simulink model "ALL_JP360_DBW_V6_5_1103"  (R2022a)
settings: Solver=FixedStepAuto  StartTime=0.0  StopTime=inf  FixedStep=0.01  RelTol=1e-3  EnableMultiTasking=on
model workspace (MAT data in the model file):
  g = 9.8
undefined symbols (not defined in the file or in its folder): canChannel, delta_v_p, IPM_Line_C0, IPM_Line_C1, IPM_Line_C2, IPM_Line_C3, M, M_p, MRR_ObjDistX, MRR_ObjDistY, MRR_ObjFusionCamID, MRR_ObjFusionSig, MRR_ObjID, MRR_ObjRelVelX, MRR_ObjRelVelY, MRR_ObjType, MRR_ObjUpdFlg, none, obj_vaild, untracktime, V, videoinput
libraries: canfdmsglib x230, canfdlib x76, slpidlib x24, simulink x18, dspstat3 x14, ctrlSharedLib x1, simulink_extras x1, imaqlib x1, realtime_pacer_lib x1, dspvision x1, visionsinks x1
(part 46 of 55)

== system ALL_JP360_DBW_V6_5_1103/MsgFromCAN/VR_ADCU_MsgFromCAN/VR_ADCU_MRR_ObjHeader_0x680 ==
  VR_ADCU_MRR_ObjHeader_0x680FromInData : Inport  OutDataTypeStr=Bus:CAN_FD_MESSAGE_BUS
  Bus Creator : BusCreator  Inputs=9  OutDataTypeStr=Bus:VR_ADCU_MRR_ObjHeader_0x680  NonVirtualBus=on
  CAN FD Unpack : canfdmsglib/CAN FD Unpack  CANdbFile=HiFire_T360_P789_1R1V_Pri_Matrix_CAN_V2.3_20220810.dbc  MsgList=(none)  MsgName=MRR_ObjHeader_0x680  ProtocolMode=CAN FD  MsgIDType=Standard (11-bit identifier)  MsgIdentifier=1664  MsgLength=20  SignalInfo={'MRR_AlignmentFail','6','1','BE','unsigned','Standard','0','1','0','0','1';'MRR_Calib_State','5','1','BE','unsigned','Standard','0','1','0','0','1';'MRR_HWFail','7','1','BE','unsigned','Standard','0','1','0','0','1';'MRR_ObjHeader_CRC','152','16','BE','unsigned','Standard','0','1','0','0','65535';'MRR_ObjHeader_MsgCounter','136','4','BE','unsigned','Standard','0','1','0','0','15';'MRR_Obj_TimeStampStatus','72','8','BE','unsigned','Standard','0','1','0','0','255';'MRR_Obj_TimeStamp_Nsec','66','30','BE','unsigned','Standard','0','1','0','0','1073741823';'MRR_Obj_TimeStamp_sec','32','32','BE','unsigned','Standard','0','1','0','0','4294967295';'MRR_Sensor_Dirty','4','1','BE','unsigned','Standard','0','1','0','0','1'}  IDPort=off  TimestampPort=off  ErrorPort=off  RemotePort=off  LengthPort=off  StatusPort=off  BRSPort=off  ESIPort=off  DLCPort=off  ApplyMinMax=off
      settings: SourceProductBaseCode=ME,XP,VN  DataFormat=CANdb specified signals
  Data Type Conversion{1..3,9} (4 alike) : DataTypeConversion  OutDataTypeStr=boolean  SaturateOnIntegerOverflow=off  RndMeth=Floor
  Data Type Conversion4 : DataTypeConversion  OutDataTypeStr=uint16  SaturateOnIntegerOverflow=off  RndMeth=Floor
  Data Type Conversion5 : DataTypeConversion  OutDataTypeStr=int8  SaturateOnIntegerOverflow=off  RndMeth=Floor
  Data Type Conversion6 : DataTypeConversion  OutDataTypeStr=uint8  SaturateOnIntegerOverflow=off  RndMeth=Floor
  Data Type Conversion7 : DataTypeConversion  OutDataTypeStr=int32  SaturateOnIntegerOverflow=off  RndMeth=Floor
  Data Type Conversion8 : DataTypeConversion  OutDataTypeStr=uint32  SaturateOnIntegerOverflow=off  RndMeth=Floor
  VR_ADCU_MRR_ObjHeader_0x680FromOutData : Outport  OutDataTypeStr=Bus:VR_ADCU_MRR_ObjHeader_0x680
  wires:
  CAN FD Unpack/1 -> Data Type Conversion1/1
  CAN FD Unpack/2 -> Data Type Conversion2/1
  CAN FD Unpack/3 -> Data Type Conversion3/1
  CAN FD Unpack/4 -> Data Type Conversion4/1
  CAN FD Unpack/5 -> Data Type Conversion5/1
  CAN FD Unpack/6 -> Data Type Conversion6/1
  CAN FD Unpack/7 -> Data Type Conversion7/1
  CAN FD Unpack/8 -> Data Type Conversion8/1
  CAN FD Unpack/9 -> Data Type Conversion9/1
  Data Type Conversion1/1 -> Bus Creator/1  "MRR_AlignmentFail"
  Data Type Conversion2/1 -> Bus Creator/2  "MRR_Calib_State"
  Data Type Conversion3/1 -> Bus Creator/3  "MRR_HWFail"
  Data Type Conversion4/1 -> Bus Creator/4  "MRR_ObjHeader_CRC"
  Data Type Conversion5/1 -> Bus Creator/5  "MRR_ObjHeader_MsgCounter"
  Data Type Conversion6/1 -> Bus Creator/6  "MRR_Obj_TimeStampStatus"
  Data Type Conversion7/1 -> Bus Creator/7  "MRR_Obj_TimeStamp_Nsec"
  Data Type Conversion8/1 -> Bus Creator/8  "MRR_Obj_TimeStamp_sec"
  Data Type Conversion9/1 -> Bus Creator/9  "MRR_Sensor_Dirty"
  Bus Creator/1 -> VR_ADCU_MRR_ObjHeader_0x680FromOutData/1  "VR_ADCU_MRR_ObjHeader_0x680FromOutData"
  VR_ADCU_MRR_ObjHeader_0x680FromInData/1 -> CAN FD Unpack/1  "VR_ADCU_MRR_ObjHeader_0x680FromInData"

== system ALL_JP360_DBW_V6_5_1103/MsgFromCAN/VR_ADCU_MsgFromCAN/VR_ADCU_MRR_Obj_01_02_0x690 ==
  VR_ADCU_MRR_Obj_01_02_0x690FromInData : Inport  OutDataTypeStr=Bus:CAN_FD_MESSAGE_BUS
  Bus Creator : BusCreator  Inputs=30  OutDataTypeStr=Bus:VR_ADCU_MRR_Obj_01_02_0x690  NonVirtualBus=on
  CAN FD Unpack : canfdmsglib/CAN FD Unpack  CANdbFile=HiFire_T360_P789_1R1V_Pri_Matrix_CAN_V2.3_20220810.dbc  MsgList=(none)  MsgName=MRR_Obj_01_02_0x690  ProtocolMode=CAN FD  MsgIDType=Standard (11-bit identifier)  MsgIdentifier=1680  MsgLength=32  SignalInfo={'MRR_ObjDistX_01','26','12','BE','unsigned','Standard','0','0.0625','0','0','254.9375';'MRR_ObjDistX_02','130','12','BE','unsigned','Standard','0','0.0625','0','0','254.9375';'MRR_ObjDistY_01','44','14','BE','unsigned','Standard','0','0.0078125','-64','-64','63.9922';'MRR_ObjDistY_02','148','14','BE','unsigned','Standard','0','0.0078125','-64','-64','63.9922';'MRR_ObjExistProb_01','11','5','BE','unsigned','Standard','0','0.03125','0','0','0.96875';'MRR_ObjExistProb_02','115','5','BE','unsigned','Standard','0','0.03125','0','0','0.96875';'MRR_ObjFusionCamID_01','208','8','BE','unsigned','Standard','0','1','0','0','255';'MRR_ObjFusionCamID_02','216','8','BE','unsigned','Standard','0','1','0','0','255';'MRR_ObjFusionSig_01','98','2','BE','unsigned','Standard','0','1','0','0','3';'MRR_ObjFusionSig_02','202','2','BE','unsigned','Standard','0','1','0','0','3';'MRR_ObjID_01','0','8','BE','unsigned','Standard','0','1','0','0','255';'MRR_ObjID_02','104','8','BE','unsigned','Standard','0','1','0','0','255';'MRR_ObjMovingSts_01','103','3','BE','unsigned','Standard','0','1','0','0','7';'MRR_ObjMovingSts_02','207','3','BE','unsigned','Standard','0','1','0','0','7';'MRR_ObjObstacleProb_01','22','5','BE','unsigned','Standard','0','0.03125','0','0','0.96875';'MRR_ObjObstacleProb_02','126','5','BE','unsigned','Standard','0','0.03125','0','0','0.96875';'MRR_ObjRelAccelX_01','72','10','BE','unsigned','Standard','0','0.03125','-16','-16','15.9688';'MRR_ObjRelAccelX_02','176','10','BE','unsigned','Standard','0','0.03125','-16','-16','15.9688';'MRR_ObjRelAccelY_01','94','10','BE','unsigned','Standard','0','0.03125','-16','-16','15.9688';'MRR_ObjRelAccelY_02','198','10','BE','unsigned','Standard','0','0.03125','-16','-16','15.9688';'MRR_ObjRelVelX_01','63','13','BE','unsigned','Standard','0','0.03125','-128','-128','127.9688';'MRR_ObjRelVelX_02','167','13','BE','unsigned','Standard','0','0.03125','-128','-128','127.9688';'MRR_ObjRelVelY_01','66','13','BE','unsigned','Standard','0','0.03125','-128','-128','127.9688';'MRR_ObjRelVelY_02','170','13','BE','unsigned','Standard','0','0.03125','-128','-128','127.9688';'MRR_ObjType_01','90','4','BE','unsigned','Standard','0','1','0','0','15';'MRR_ObjType_02','194','4','BE','unsigned','Standard','0','1','0','0','15';'MRR_ObjUpdFlg_01','100','3','BE','unsigned','Standard','0','1','0','0','7';'MRR_ObjUpdFlg_02','204','3','BE','unsigned','Standard','0','1','0','0','7';'MRR_Obj_01_02_Checksum','248','16','BE','unsigned','Standard','0','1','0','0','65535';'MRR_Obj_01_02_MsgCounter','232','4','BE','unsigned','Standard','0','1','0','0','15'}  IDPort=off  TimestampPort=off  ErrorPort=off  RemotePort=off  LengthPort=off  StatusPort=off  BRSPort=off  ESIPort=off  DLCPort=off  ApplyMinMax=off
      settings: SourceProductBaseCode=ME,XP,VN  DataFormat=CANdb specified signals
  Data Type Conversion{1..6,15..24} (16 alike) : DataTypeConversion  OutDataTypeStr=single  SaturateOnIntegerOverflow=off  RndMeth=Floor
  Data Type Conversion{9..10,13..14,25..28,30} (9 alike) : DataTypeConversion  OutDataTypeStr=int8  SaturateOnIntegerOverflow=off  RndMeth=Floor
  Data Type Conversion{7..8,11..12} (4 alike) : DataTypeConversion  OutDataTypeStr=uint8  SaturateOnIntegerOverflow=off  RndMeth=Floor
  Data Type Conversion29 : DataTypeConversion  OutDataTypeStr=uint16  SaturateOnIntegerOverflow=off  RndMeth=Floor
  VR_ADCU_MRR_Obj_01_02_0x690FromOutData : Outport  OutDataTypeStr=Bus:VR_ADCU_MRR_Obj_01_02_0x690
  wires:
  CAN FD Unpack/1 -> Data Type Conversion1/1
  CAN FD Unpack/2 -> Data Type Conversion2/1
  CAN FD Unpack/3 -> Data Type Conversion3/1
  CAN FD Unpack/4 -> Data Type Conversion4/1
  CAN FD Unpack/5 -> Data Type Conversion5/1
  CAN FD Unpack/6 -> Data Type Conversion6/1
  CAN FD Unpack/7 -> Data Type Conversion7/1
  CAN FD Unpack/8 -> Data Type Conversion8/1
  CAN FD Unpack/9 -> Data Type Conversion9/1
  CAN FD Unpack/10 -> Data Type Conversion10/1
  CAN FD Unpack/11 -> Data Type Conversion11/1
  CAN FD Unpack/12 -> Data Type Conversion12/1
  CAN FD Unpack/13 -> Data Type Conversion13/1
  CAN FD Unpack/14 -> Data Type Conversion14/1
  CAN FD Unpack/15 -> Data Type Conversion15/1
  CAN FD Unpack/16 -> Data Type Conversion16/1
  CAN FD Unpack/17 -> Data Type Conversion17/1
  CAN FD Unpack/18 -> Data Type Conversion18/1
  CAN FD Unpack/19 -> Data Type Conversion19/1
  CAN FD Unpack/20 -> Data Type Conversion20/1
  CAN FD Unpack/21 -> Data Type Conversion21/1
  CAN FD Unpack/22 -> Data Type Conversion22/1
  CAN FD Unpack/23 -> Data Type Conversion23/1
  CAN FD Unpack/24 -> Data Type Conversion24/1
  CAN FD Unpack/25 -> Data Type Conversion25/1
  CAN FD Unpack/26 -> Data Type Conversion26/1
  CAN FD Unpack/27 -> Data Type Conversion27/1
  CAN FD Unpack/28 -> Data Type Conversion28/1
  CAN FD Unpack/29 -> Data Type Conversion29/1
  CAN FD Unpack/30 -> Data Type Conversion30/1
  Data Type Conversion1/1 -> Bus Creator/1  "MRR_ObjDistX_01"
  Data Type Conversion2/1 -> Bus Creator/2  "MRR_ObjDistX_02"
  Data Type Conversion3/1 -> Bus Creator/3  "MRR_ObjDistY_01"
  Data Type Conversion4/1 -> Bus Creator/4  "MRR_ObjDistY_02"
  Data Type Conversion5/1 -> Bus Creator/5  "MRR_ObjExistProb_01"
  Data Type Conversion6/1 -> Bus Creator/6  "MRR_ObjExistProb_02"
  Data Type Conversion7/1 -> Bus Creator/7  "MRR_ObjFusionCamID_01"
  Data Type Conversion8/1 -> Bus Creator/8  "MRR_ObjFusionCamID_02"
  Data Type Conversion9/1 -> Bus Creator/9  "MRR_ObjFusionSig_01"
  Data Type Conversion10/1 -> Bus Creator/10  "MRR_ObjFusionSig_02"
  Data Type Conversion11/1 -> Bus Creator/11  "MRR_ObjID_01"
  Data Type Conversion12/1 -> Bus Creator/12  "MRR_ObjID_02"
  Data Type Conversion13/1 -> Bus Creator/13  "MRR_ObjMovingSts_01"
  Data Type Conversion14/1 -> Bus Creator/14  "MRR_ObjMovingSts_02"
  Data Type Conversion15/1 -> Bus Creator/15  "MRR_ObjObstacleProb_01"
  Data Type Conversion16/1 -> Bus Creator/16  "MRR_ObjObstacleProb_02"
  Data Type Conversion17/1 -> Bus Creator/17  "MRR_ObjRelAccelX_01"
  Data Type Conversion18/1 -> Bus Creator/18  "MRR_ObjRelAccelX_02"
  Data Type Conversion19/1 -> Bus Creator/19  "MRR_ObjRelAccelY_01"
  Data Type Conversion20/1 -> Bus Creator/20  "MRR_ObjRelAccelY_02"
  Data Type Conversion21/1 -> Bus Creator/21  "MRR_ObjRelVelX_01"
  Data Type Conversion22/1 -> Bus Creator/22  "MRR_ObjRelVelX_02"
  Data Type Conversion23/1 -> Bus Creator/23  "MRR_ObjRelVelY_01"
  Data Type Conversion24/1 -> Bus Creator/24  "MRR_ObjRelVelY_02"
  Data Type Conversion25/1 -> Bus Creator/25  "MRR_ObjType_01"
  Data Type Conversion26/1 -> Bus Creator/26  "MRR_ObjType_02"
  Data Type Conversion27/1 -> Bus Creator/27  "MRR_ObjUpdFlg_01"
  Data Type Conversion28/1 -> Bus Creator/28  "MRR_ObjUpdFlg_02"
  Data Type Conversion29/1 -> Bus Creator/29  "MRR_Obj_01_02_Checksum"
  Data Type Conversion30/1 -> Bus Creator/30  "MRR_Obj_01_02_MsgCounter"
  Bus Creator/1 -> VR_ADCU_MRR_Obj_01_02_0x690FromOutData/1  "VR_ADCU_MRR_Obj_01_02_0x690FromOutData"
  VR_ADCU_MRR_Obj_01_02_0x690FromInData/1 -> CAN FD Unpack/1  "VR_ADCU_MRR_Obj_01_02_0x690FromInData"

== system ALL_JP360_DBW_V6_5_1103/MsgFromCAN/VR_ADCU_MsgFromCAN/VR_ADCU_MRR_Obj_03_04_0x691 ==
  VR_ADCU_MRR_Obj_03_04_0x691FromInData : Inport  OutDataTypeStr=Bus:CAN_FD_MESSAGE_BUS
  Bus Creator : BusCreator  Inputs=30  OutDataTypeStr=Bus:VR_ADCU_MRR_Obj_03_04_0x691  NonVirtualBus=on
  CAN FD Unpack : canfdmsglib/CAN FD Unpack  CANdbFile=HiFire_T360_P789_1R1V_Pri_Matrix_CAN_V2.3_20220810.dbc  MsgList=(none)  MsgName=MRR_Obj_03_04_0x691  ProtocolMode=CAN FD  MsgIDType=Standard (11-bit identifier)  MsgIdentifier=1681  MsgLength=32  SignalInfo={'MRR_ObjDistX_03','26','12','BE','unsigned','Standard','0','0.0625','0','0','254.9375';'MRR_ObjDistX_04','130','12','BE','unsigned','Standard','0','0.0625','0','0','254.9375';'MRR_ObjDistY_03','44','14','BE','unsigned','Standard','0','0.0078125','-64','-64','63.9922';'MRR_ObjDistY_04','148','14','BE','unsigned','Standard','0','0.0078125','-64','-64','63.9922';'MRR_ObjExistProb_03','11','5','BE','unsigned','Standard','0','0.03125','0','0','0.96875';'MRR_ObjExistProb_04','115','5','BE','unsigned','Standard','0','0.03125','0','0','0.96875';'MRR_ObjFusionCamID_03','208','8','BE','unsigned','Standard','0','1','0','0','255';'MRR_ObjFusionCamID_04','216','8','BE','unsigned','Standard','0','1','0','0','255';'MRR_ObjFusionSig_03','98','2','BE','unsigned','Standard','0','1','0','0','3';'MRR_ObjFusionSig_04','202','2','BE','unsigned','Standard','0','1','0','0','3';'MRR_ObjID_03','0','8','BE','unsigned','Standard','0','1','0','0','255';'MRR_ObjID_04','104','8','BE','unsigned','Standard','0','1','0','0','255';'MRR_ObjMovingSts_03','103','3','BE','unsigned','Standard','0','1','0','0','7';'MRR_ObjMovingSts_04','207','3','BE','unsigned','Standard','0','1','0','0','7';'MRR_ObjObstacleProb_03','22','5','BE','unsigned','Standard','0','0.03125','0','0','0.96875';'MRR_ObjObstacleProb_04','126','5','BE','unsigned','Standard','0','0.03125','0','0','0.96875';'MRR_ObjRelAccelX_03','72','10','BE','unsigned','Standard','0','0.03125','-16','-16','15.9688';'MRR_ObjRelAccelX_04','176','10','BE','unsigned','Standard','0','0.03125','-16','-16','15.9688';'MRR_ObjRelAccelY_03','94','10','BE','unsigned','Standard','0','0.03125','-16','-16','15.9688';'MRR_ObjRelAccelY_04','198','10','BE','unsigned','Standard','0','0.03125','-16','-16','15.9688';'MRR_ObjRelVelX_03','63','13','BE','unsigned','Standard','0','0.03125','-128','-128','127.9688';'MRR_ObjRelVelX_04','167','13','BE','unsigned','Standard','0','0.03125','-128','-128','127.9688';'MRR_ObjRelVelY_03','66','13','BE','unsigned','Standard','0','0.03125','-128','-128','127.9688';'MRR_ObjRelVelY_04','170','13','BE','unsigned','Standard','0','0.03125','-128','-128','127.9688';'MRR_ObjType_03','90','4','BE','unsigned','Standard','0','1','0','0','15';'MRR_ObjType_04','194','4','BE','unsigned','Standard','0','1','0','0','15';'MRR_ObjUpdFlg_03','100','3','BE','unsigned','Standard','0','1','0','0','7';'MRR_ObjUpdFlg_04','204','3','BE','unsigned','Standard','0','1','0','0','7';'MRR_Obj_03_04_Checksum','248','16','BE','unsigned','Standard','0','1','0','0','65535';'MRR_Obj_03_04_MsgCounter','232','4','BE','unsigned','Standard','0','1','0','0','15'}  IDPort=off  TimestampPort=off  ErrorPort=off  RemotePort=off  LengthPort=off  StatusPort=off  BRSPort=off  ESIPort=off  DLCPort=off  ApplyMinMax=off
      settings: SourceProductBaseCode=ME,XP,VN  DataFormat=CANdb specified signals
  Data Type Conversion{1..6,15..24} (16 alike) : DataTypeConversion  OutDataTypeStr=single  SaturateOnIntegerOverflow=off  RndMeth=Floor
  Data Type Conversion{9..10,13..14,25..28,30} (9 alike) : DataTypeConversion  OutDataTypeStr=int8  SaturateOnIntegerOverflow=off  RndMeth=Floor
  Data Type Conversion{7..8,11..12} (4 alike) : DataTypeConversion  OutDataTypeStr=uint8  SaturateOnIntegerOverflow=off  RndMeth=Floor
  Data Type Conversion29 : DataTypeConversion  OutDataTypeStr=uint16  SaturateOnIntegerOverflow=off  RndMeth=Floor
  VR_ADCU_MRR_Obj_03_04_0x691FromOutData : Outport  OutDataTypeStr=Bus:VR_ADCU_MRR_Obj_03_04_0x691
  wires:
  CAN FD Unpack/1 -> Data Type Conversion1/1
  CAN FD Unpack/2 -> Data Type Conversion2/1
  CAN FD Unpack/3 -> Data Type Conversion3/1
  CAN FD Unpack/4 -> Data Type Conversion4/1
  CAN FD Unpack/5 -> Data Type Conversion5/1
  CAN FD Unpack/6 -> Data Type Conversion6/1
  CAN FD Unpack/7 -> Data Type Conversion7/1
  CAN FD Unpack/8 -> Data Type Conversion8/1
  CAN FD Unpack/9 -> Data Type Conversion9/1
  CAN FD Unpack/10 -> Data Type Conversion10/1
  CAN FD Unpack/11 -> Data Type Conversion11/1
  CAN FD Unpack/12 -> Data Type Conversion12/1
  CAN FD Unpack/13 -> Data Type Conversion13/1
  CAN FD Unpack/14 -> Data Type Conversion14/1
  CAN FD Unpack/15 -> Data Type Conversion15/1
  CAN FD Unpack/16 -> Data Type Conversion16/1
  CAN FD Unpack/17 -> Data Type Conversion17/1
  CAN FD Unpack/18 -> Data Type Conversion18/1
  CAN FD Unpack/19 -> Data Type Conversion19/1
  CAN FD Unpack/20 -> Data Type Conversion20/1
  CAN FD Unpack/21 -> Data Type Conversion21/1
  CAN FD Unpack/22 -> Data Type Conversion22/1
  CAN FD Unpack/23 -> Data Type Conversion23/1
  CAN FD Unpack/24 -> Data Type Conversion24/1
  CAN FD Unpack/25 -> Data Type Conversion25/1
  CAN FD Unpack/26 -> Data Type Conversion26/1
  CAN FD Unpack/27 -> Data Type Conversion27/1
  CAN FD Unpack/28 -> Data Type Conversion28/1
  CAN FD Unpack/29 -> Data Type Conversion29/1
  CAN FD Unpack/30 -> Data Type Conversion30/1
  Data Type Conversion1/1 -> Bus Creator/1  "MRR_ObjDistX_03"
  Data Type Conversion2/1 -> Bus Creator/2  "MRR_ObjDistX_04"
  Data Type Conversion3/1 -> Bus Creator/3  "MRR_ObjDistY_03"
  Data Type Conversion4/1 -> Bus Creator/4  "MRR_ObjDistY_04"
  Data Type Conversion5/1 -> Bus Creator/5  "MRR_ObjExistProb_03"
  Data Type Conversion6/1 -> Bus Creator/6  "MRR_ObjExistProb_04"
  Data Type Conversion7/1 -> Bus Creator/7  "MRR_ObjFusionCamID_03"
  Data Type Conversion8/1 -> Bus Creator/8  "MRR_ObjFusionCamID_04"
  Data Type Conversion9/1 -> Bus Creator/9  "MRR_ObjFusionSig_03"
  Data Type Conversion10/1 -> Bus Creator/10  "MRR_ObjFusionSig_04"
  Data Type Conversion11/1 -> Bus Creator/11  "MRR_ObjID_03"
  Data Type Conversion12/1 -> Bus Creator/12  "MRR_ObjID_04"
  Data Type Conversion13/1 -> Bus Creator/13  "MRR_ObjMovingSts_03"
  Data Type Conversion14/1 -> Bus Creator/14  "MRR_ObjMovingSts_04"
  Data Type Conversion15/1 -> Bus Creator/15  "MRR_ObjObstacleProb_03"
  Data Type Conversion16/1 -> Bus Creator/16  "MRR_ObjObstacleProb_04"
  Data Type Conversion17/1 -> Bus Creator/17  "MRR_ObjRelAccelX_03"
  Data Type Conversion18/1 -> Bus Creator/18  "MRR_ObjRelAccelX_04"
  Data Type Conversion19/1 -> Bus Creator/19  "MRR_ObjRelAccelY_03"
  Data Type Conversion20/1 -> Bus Creator/20  "MRR_ObjRelAccelY_04"
  Data Type Conversion21/1 -> Bus Creator/21  "MRR_ObjRelVelX_03"
  Data Type Conversion22/1 -> Bus Creator/22  "MRR_ObjRelVelX_04"
  Data Type Conversion23/1 -> Bus Creator/23  "MRR_ObjRelVelY_03"
  Data Type Conversion24/1 -> Bus Creator/24  "MRR_ObjRelVelY_04"
  Data Type Conversion25/1 -> Bus Creator/25  "MRR_ObjType_03"
  Data Type Conversion26/1 -> Bus Creator/26  "MRR_ObjType_04"
  Data Type Conversion27/1 -> Bus Creator/27  "MRR_ObjUpdFlg_03"
  Data Type Conversion28/1 -> Bus Creator/28  "MRR_ObjUpdFlg_04"
  Data Type Conversion29/1 -> Bus Creator/29  "MRR_Obj_03_04_Checksum"
  Data Type Conversion30/1 -> Bus Creator/30  "MRR_Obj_03_04_MsgCounter"
  Bus Creator/1 -> VR_ADCU_MRR_Obj_03_04_0x691FromOutData/1  "VR_ADCU_MRR_Obj_03_04_0x691FromOutData"
  VR_ADCU_MRR_Obj_03_04_0x691FromInData/1 -> CAN FD Unpack/1  "VR_ADCU_MRR_Obj_03_04_0x691FromInData"

== system ALL_JP360_DBW_V6_5_1103/MsgFromCAN/VR_ADCU_MsgFromCAN/VR_ADCU_MRR_Obj_05_06_0x692 ==
  VR_ADCU_MRR_Obj_05_06_0x692FromInData : Inport  OutDataTypeStr=Bus:CAN_FD_MESSAGE_BUS
  Bus Creator : BusCreator  Inputs=30  OutDataTypeStr=Bus:VR_ADCU_MRR_Obj_05_06_0x692  NonVirtualBus=on
  CAN FD Unpack : canfdmsglib/CAN FD Unpack  CANdbFile=HiFire_T360_P789_1R1V_Pri_Matrix_CAN_V2.3_20220810.dbc  MsgList=(none)  MsgName=MRR_Obj_05_06_0x692  ProtocolMode=CAN FD  MsgIDType=Standard (11-bit identifier)  MsgIdentifier=1682  MsgLength=32  SignalInfo={'MRR_ObjDistX_05','26','12','BE','unsigned','Standard','0','0.0625','0','0','254.9375';'MRR_ObjDistX_06','130','12','BE','unsigned','Standard','0','0.0625','0','0','254.9375';'MRR_ObjDistY_05','44','14','BE','unsigned','Standard','0','0.0078125','-64','-64','63.9922';'MRR_ObjDistY_06','148','14','BE','unsigned','Standard','0','0.0078125','-64','-64','63.9922';'MRR_ObjExistProb_05','11','5','BE','unsigned','Standard','0','0.03125','0','0','0.96875';'MRR_ObjExistProb_06','115','5','BE','unsigned','Standard','0','0.03125','0','0','0.96875';'MRR_ObjFusionCamID_05','208','8','BE','unsigned','Standard','0','1','0','0','255';'MRR_ObjFusionCamID_06','216','8','BE','unsigned','Standard','0','1','0','0','255';'MRR_ObjFusionSig_05','98','2','BE','unsigned','Standard','0','1','0','0','3';'MRR_ObjFusionSig_06','202','2','BE','unsigned','Standard','0','1','0','0','3';'MRR_ObjID_05','0','8','BE','unsigned','Standard','0','1','0','0','255';'MRR_ObjID_06','104','8','BE','unsigned','Standard','0','1','0','0','255';'MRR_ObjMovingSts_05','103','3','BE','unsigned','Standard','0','1','0','0','7';'MRR_ObjMovingSts_06','207','3','BE','unsigned','Standard','0','1','0','0','7';'MRR_ObjObstacleProb_05','22','5','BE','unsigned','Standard','0','0.03125','0','0','0.96875';'MRR_ObjObstacleProb_06','126','5','BE','unsigned','Standard','0','0.03125','0','0','0.96875';'MRR_ObjRelAccelX_05','72','10','BE','unsigned','Standard','0','0.03125','-16','-16','15.9688';'MRR_ObjRelAccelX_06','176','10','BE','unsigned','Standard','0','0.03125','-16','-16','15.9688';'MRR_ObjRelAccelY_05','94','10','BE','unsigned','Standard','0','0.03125','-16','-16','15.9688';'MRR_ObjRelAccelY_06','198','10','BE','unsigned','Standard','0','0.03125','-16','-16','15.9688';'MRR_ObjRelVelX_05','63','13','BE','unsigned','Standard','0','0.03125','-128','-128','127.9688';'MRR_ObjRelVelX_06','167','13','BE','unsigned','Standard','0','0.03125','-128','-128','127.9688';'MRR_ObjRelVelY_05','66','13','BE','unsigned','Standard','0','0.03125','-128','-128','127.9688';'MRR_ObjRelVelY_06','170','13','BE','unsigned','Standard','0','0.03125','-128','-128','127.9688';'MRR_ObjType_05','90','4','BE','unsigned','Standard','0','1','0','0','15';'MRR_ObjType_06','194','4','BE','unsigned','Standard','0','1','0','0','15';'MRR_ObjUpdFlg_05','100','3','BE','unsigned','Standard','0','1','0','0','7';'MRR_ObjUpdFlg_06','204','3','BE','unsigned','Standard','0','1','0','0','7';'MRR_Obj_05_06_Checksum','248','16','BE','unsigned','Standard','0','1','0','0','65535';'MRR_Obj_05_06_MsgCounter','232','4','BE','unsigned','Standard','0','1','0','0','15'}  IDPort=off  TimestampPort=off  ErrorPort=off  RemotePort=off  LengthPort=off  StatusPort=off  BRSPort=off  ESIPort=off  DLCPort=off  ApplyMinMax=off
      settings: SourceProductBaseCode=ME,XP,VN  DataFormat=CANdb specified signals
  Data Type Conversion{1..6,15..24} (16 alike) : DataTypeConversion  OutDataTypeStr=single  SaturateOnIntegerOverflow=off  RndMeth=Floor
  Data Type Conversion{9..10,13..14,25..28,30} (9 alike) : DataTypeConversion  OutDataTypeStr=int8  SaturateOnIntegerOverflow=off  RndMeth=Floor
  Data Type Conversion{7..8,11..12} (4 alike) : DataTypeConversion  OutDataTypeStr=uint8  SaturateOnIntegerOverflow=off  RndMeth=Floor
  Data Type Conversion29 : DataTypeConversion  OutDataTypeStr=uint16  SaturateOnIntegerOverflow=off  RndMeth=Floor
  VR_ADCU_MRR_Obj_05_06_0x692FromOutData : Outport  OutDataTypeStr=Bus:VR_ADCU_MRR_Obj_05_06_0x692
  wires:
  CAN FD Unpack/1 -> Data Type Conversion1/1
  CAN FD Unpack/2 -> Data Type Conversion2/1
  CAN FD Unpack/3 -> Data Type Conversion3/1
  CAN FD Unpack/4 -> Data Type Conversion4/1
  CAN FD Unpack/5 -> Data Type Conversion5/1
  CAN FD Unpack/6 -> Data Type Conversion6/1
  CAN FD Unpack/7 -> Data Type Conversion7/1
  CAN FD Unpack/8 -> Data Type Conversion8/1
  CAN FD Unpack/9 -> Data Type Conversion9/1
  CAN FD Unpack/10 -> Data Type Conversion10/1
  CAN FD Unpack/11 -> Data Type Conversion11/1
  CAN FD Unpack/12 -> Data Type Conversion12/1
  CAN FD Unpack/13 -> Data Type Conversion13/1
  CAN FD Unpack/14 -> Data Type Conversion14/1
  CAN FD Unpack/15 -> Data Type Conversion15/1
  CAN FD Unpack/16 -> Data Type Conversion16/1
  CAN FD Unpack/17 -> Data Type Conversion17/1
  CAN FD Unpack/18 -> Data Type Conversion18/1
  CAN FD Unpack/19 -> Data Type Conversion19/1
  CAN FD Unpack/20 -> Data Type Conversion20/1
  CAN FD Unpack/21 -> Data Type Conversion21/1
  CAN FD Unpack/22 -> Data Type Conversion22/1
  CAN FD Unpack/23 -> Data Type Conversion23/1
  CAN FD Unpack/24 -> Data Type Conversion24/1
  CAN FD Unpack/25 -> Data Type Conversion25/1
  CAN FD Unpack/26 -> Data Type Conversion26/1
  CAN FD Unpack/27 -> Data Type Conversion27/1
  CAN FD Unpack/28 -> Data Type Conversion28/1
  CAN FD Unpack/29 -> Data Type Conversion29/1
  CAN FD Unpack/30 -> Data Type Conversion30/1
  Data Type Conversion1/1 -> Bus Creator/1  "MRR_ObjDistX_05"
  Data Type Conversion2/1 -> Bus Creator/2  "MRR_ObjDistX_06"
  Data Type Conversion3/1 -> Bus Creator/3  "MRR_ObjDistY_05"
  Data Type Conversion4/1 -> Bus Creator/4  "MRR_ObjDistY_06"
  Data Type Conversion5/1 -> Bus Creator/5  "MRR_ObjExistProb_05"
  Data Type Conversion6/1 -> Bus Creator/6  "MRR_ObjExistProb_06"
  Data Type Conversion7/1 -> Bus Creator/7  "MRR_ObjFusionCamID_05"
  Data Type Conversion8/1 -> Bus Creator/8  "MRR_ObjFusionCamID_06"
  Data Type Conversion9/1 -> Bus Creator/9  "MRR_ObjFusionSig_05"
  Data Type Conversion10/1 -> Bus Creator/10  "MRR_ObjFusionSig_06"
  Data Type Conversion11/1 -> Bus Creator/11  "MRR_ObjID_05"
  Data Type Conversion12/1 -> Bus Creator/12  "MRR_ObjID_06"
  Data Type Conversion13/1 -> Bus Creator/13  "MRR_ObjMovingSts_05"
  Data Type Conversion14/1 -> Bus Creator/14  "MRR_ObjMovingSts_06"
  Data Type Conversion15/1 -> Bus Creator/15  "MRR_ObjObstacleProb_05"
  Data Type Conversion16/1 -> Bus Creator/16  "MRR_ObjObstacleProb_06"
  Data Type Conversion17/1 -> Bus Creator/17  "MRR_ObjRelAccelX_05"
  Data Type Conversion18/1 -> Bus Creator/18  "MRR_ObjRelAccelX_06"
  Data Type Conversion19/1 -> Bus Creator/19  "MRR_ObjRelAccelY_05"
  Data Type Conversion20/1 -> Bus Creator/20  "MRR_ObjRelAccelY_06"
  Data Type Conversion21/1 -> Bus Creator/21  "MRR_ObjRelVelX_05"
  Data Type Conversion22/1 -> Bus Creator/22  "MRR_ObjRelVelX_06"
  Data Type Conversion23/1 -> Bus Creator/23  "MRR_ObjRelVelY_05"
  Data Type Conversion24/1 -> Bus Creator/24  "MRR_ObjRelVelY_06"
  Data Type Conversion25/1 -> Bus Creator/25  "MRR_ObjType_05"
  Data Type Conversion26/1 -> Bus Creator/26  "MRR_ObjType_06"
  Data Type Conversion27/1 -> Bus Creator/27  "MRR_ObjUpdFlg_05"
  Data Type Conversion28/1 -> Bus Creator/28  "MRR_ObjUpdFlg_06"
  Data Type Conversion29/1 -> Bus Creator/29  "MRR_Obj_05_06_Checksum"
  Data Type Conversion30/1 -> Bus Creator/30  "MRR_Obj_05_06_MsgCounter"
  Bus Creator/1 -> VR_ADCU_MRR_Obj_05_06_0x692FromOutData/1  "VR_ADCU_MRR_Obj_05_06_0x692FromOutData"
  VR_ADCU_MRR_Obj_05_06_0x692FromInData/1 -> CAN FD Unpack/1  "VR_ADCU_MRR_Obj_05_06_0x692FromInData"

== system ALL_JP360_DBW_V6_5_1103/MsgFromCAN/VR_ADCU_MsgFromCAN/VR_ADCU_MRR_Obj_07_08_0x693 ==
  VR_ADCU_MRR_Obj_07_08_0x693FromInData : Inport  OutDataTypeStr=Bus:CAN_FD_MESSAGE_BUS
  Bus Creator : BusCreator  Inputs=30  OutDataTypeStr=Bus:VR_ADCU_MRR_Obj_07_08_0x693  NonVirtualBus=on
  CAN FD Unpack : canfdmsglib/CAN FD Unpack  CANdbFile=HiFire_T360_P789_1R1V_Pri_Matrix_CAN_V2.3_20220810.dbc  MsgList=(none)  MsgName=MRR_Obj_07_08_0x693  ProtocolMode=CAN FD  MsgIDType=Standard (11-bit identifier)  MsgIdentifier=1683  MsgLength=32  SignalInfo={'MRR_ObjDistX_07','26','12','BE','unsigned','Standard','0','0.0625','0','0','254.9375';'MRR_ObjDistX_08','130','12','BE','unsigned','Standard','0','0.0625','0','0','254.9375';'MRR_ObjDistY_07','44','14','BE','unsigned','Standard','0','0.0078125','-64','-64','63.9922';'MRR_ObjDistY_08','148','14','BE','unsigned','Standard','0','0.0078125','-64','-64','63.9922';'MRR_ObjExistProb_07','11','5','BE','unsigned','Standard','0','0.03125','0','0','0.96875';'MRR_ObjExistProb_08','115','5','BE','unsigned','Standard','0','0.03125','0','0','0.96875';'MRR_ObjFusionCamID_07','208','8','BE','unsigned','Standard','0','1','0','0','255';'MRR_ObjFusionCamID_08','216','8','BE','unsigned','Standard','0','1','0','0','255';'MRR_ObjFusionSig_07','98','2','BE','unsigned','Standard','0','1','0','0','3';'MRR_ObjFusionSig_08','202','2','BE','unsigned','Standard','0','1','0','0','3';'MRR_ObjID_07','0','8','BE','unsigned','Standard','0','1','0','0','255';'MRR_ObjID_08','104','8','BE','unsigned','Standard','0','1','0','0','255';'MRR_ObjMovingSts_07','103','3','BE','unsigned','Standard','0','1','0','0','7';'MRR_ObjMovingSts_08','207','3','BE','unsigned','Standard','0','1','0','0','7';'MRR_ObjObstacleProb_07','22','5','BE','unsigned','Standard','0','0.03125','0','0','0.96875';'MRR_ObjObstacleProb_08','126','5','BE','unsigned','Standard','0','0.03125','0','0','0.96875';'MRR_ObjRelAccelX_07','72','10','BE','unsigned','Standard','0','0.03125','-16','-16','15.9688';'MRR_ObjRelAccelX_08','176','10','BE','unsigned','Standard','0','0.03125','-16','-16','15.9688';'MRR_ObjRelAccelY_07','94','10','BE','unsigned','Standard','0','0.03125','-16','-16','15.9688';'MRR_ObjRelAccelY_08','198','10','BE','unsigned','Standard','0','0.03125','-16','-16','15.9688';'MRR_ObjRelVelX_07','63','13','BE','unsigned','Standard','0','0.03125','-128','-128','127.9688';'MRR_ObjRelVelX_08','167','13','BE','unsigned','Standard','0','0.03125','-128','-128','127.9688';'MRR_ObjRelVelY_07','66','13','BE','unsigned','Standard','0','0.03125','-128','-128','127.9688';'MRR_ObjRelVelY_08','170','13','BE','unsigned','Standard','0','0.03125','-128','-128','127.9688';'MRR_ObjType_07','90','4','BE','unsigned','Standard','0','1','0','0','15';'MRR_ObjType_08','194','4','BE','unsigned','Standard','0','1','0','0','15';'MRR_ObjUpdFlg_07','100','3','BE','unsigned','Standard','0','1','0','0','7';'MRR_ObjUpdFlg_08','204','3','BE','unsigned','Standard','0','1','0','0','7';'MRR_Obj_07_08_Checksum','248','16','BE','unsigned','Standard','0','1','0','0','65535';'MRR_Obj_07_08_MsgCounter','232','4','BE','unsigned','Standard','0','1','0','0','15'}  IDPort=off  TimestampPort=off  ErrorPort=off  RemotePort=off  LengthPort=off  StatusPort=off  BRSPort=off  ESIPort=off  DLCPort=off  ApplyMinMax=off
      settings: SourceProductBaseCode=ME,XP,VN  DataFormat=CANdb specified signals
  Data Type Conversion{1..6,15..24} (16 alike) : DataTypeConversion  OutDataTypeStr=single  SaturateOnIntegerOverflow=off  RndMeth=Floor
  Data Type Conversion{9..10,13..14,25..28,30} (9 alike) : DataTypeConversion  OutDataTypeStr=int8  SaturateOnIntegerOverflow=off  RndMeth=Floor
  Data Type Conversion{7..8,11..12} (4 alike) : DataTypeConversion  OutDataTypeStr=uint8  SaturateOnIntegerOverflow=off  RndMeth=Floor
  Data Type Conversion29 : DataTypeConversion  OutDataTypeStr=uint16  SaturateOnIntegerOverflow=off  RndMeth=Floor
  VR_ADCU_MRR_Obj_07_08_0x693FromOutData : Outport  OutDataTypeStr=Bus:VR_ADCU_MRR_Obj_07_08_0x693
  wires:
  CAN FD Unpack/1 -> Data Type Conversion1/1
  CAN FD Unpack/2 -> Data Type Conversion2/1
  CAN FD Unpack/3 -> Data Type Conversion3/1
  CAN FD Unpack/4 -> Data Type Conversion4/1
  CAN FD Unpack/5 -> Data Type Conversion5/1
  CAN FD Unpack/6 -> Data Type Conversion6/1
  CAN FD Unpack/7 -> Data Type Conversion7/1
  CAN FD Unpack/8 -> Data Type Conversion8/1
  CAN FD Unpack/9 -> Data Type Conversion9/1
  CAN FD Unpack/10 -> Data Type Conversion10/1
  CAN FD Unpack/11 -> Data Type Conversion11/1
  CAN FD Unpack/12 -> Data Type Conversion12/1
  CAN FD Unpack/13 -> Data Type Conversion13/1
  CAN FD Unpack/14 -> Data Type Conversion14/1
  CAN FD Unpack/15 -> Data Type Conversion15/1
  CAN FD Unpack/16 -> Data Type Conversion16/1
  CAN FD Unpack/17 -> Data Type Conversion17/1
  CAN FD Unpack/18 -> Data Type Conversion18/1
  CAN FD Unpack/19 -> Data Type Conversion19/1
  CAN FD Unpack/20 -> Data Type Conversion20/1
  CAN FD Unpack/21 -> Data Type Conversion21/1
  CAN FD Unpack/22 -> Data Type Conversion22/1
  CAN FD Unpack/23 -> Data Type Conversion23/1
  CAN FD Unpack/24 -> Data Type Conversion24/1
  CAN FD Unpack/25 -> Data Type Conversion25/1
  CAN FD Unpack/26 -> Data Type Conversion26/1
  CAN FD Unpack/27 -> Data Type Conversion27/1
  CAN FD Unpack/28 -> Data Type Conversion28/1
  CAN FD Unpack/29 -> Data Type Conversion29/1
  CAN FD Unpack/30 -> Data Type Conversion30/1
  Data Type Conversion1/1 -> Bus Creator/1  "MRR_ObjDistX_07"
  Data Type Conversion2/1 -> Bus Creator/2  "MRR_ObjDistX_08"
  Data Type Conversion3/1 -> Bus Creator/3  "MRR_ObjDistY_07"
  Data Type Conversion4/1 -> Bus Creator/4  "MRR_ObjDistY_08"
  Data Type Conversion5/1 -> Bus Creator/5  "MRR_ObjExistProb_07"
  Data Type Conversion6/1 -> Bus Creator/6  "MRR_ObjExistProb_08"
  Data Type Conversion7/1 -> Bus Creator/7  "MRR_ObjFusionCamID_07"
  Data Type Conversion8/1 -> Bus Creator/8  "MRR_ObjFusionCamID_08"
  Data Type Conversion9/1 -> Bus Creator/9  "MRR_ObjFusionSig_07"
  Data Type Conversion10/1 -> Bus Creator/10  "MRR_ObjFusionSig_08"
  Data Type Conversion11/1 -> Bus Creator/11  "MRR_ObjID_07"
  Data Type Conversion12/1 -> Bus Creator/12  "MRR_ObjID_08"
  Data Type Conversion13/1 -> Bus Creator/13  "MRR_ObjMovingSts_07"
  Data Type Conversion14/1 -> Bus Creator/14  "MRR_ObjMovingSts_08"
  Data Type Conversion15/1 -> Bus Creator/15  "MRR_ObjObstacleProb_07"
  Data Type Conversion16/1 -> Bus Creator/16  "MRR_ObjObstacleProb_08"
  Data Type Conversion17/1 -> Bus Creator/17  "MRR_ObjRelAccelX_07"
  Data Type Conversion18/1 -> Bus Creator/18  "MRR_ObjRelAccelX_08"
  Data Type Conversion19/1 -> Bus Creator/19  "MRR_ObjRelAccelY_07"
  Data Type Conversion20/1 -> Bus Creator/20  "MRR_ObjRelAccelY_08"
  Data Type Conversion21/1 -> Bus Creator/21  "MRR_ObjRelVelX_07"
  Data Type Conversion22/1 -> Bus Creator/22  "MRR_ObjRelVelX_08"
  Data Type Conversion23/1 -> Bus Creator/23  "MRR_ObjRelVelY_07"
  Data Type Conversion24/1 -> Bus Creator/24  "MRR_ObjRelVelY_08"
  Data Type Conversion25/1 -> Bus Creator/25  "MRR_ObjType_07"
  Data Type Conversion26/1 -> Bus Creator/26  "MRR_ObjType_08"
  Data Type Conversion27/1 -> Bus Creator/27  "MRR_ObjUpdFlg_07"
  Data Type Conversion28/1 -> Bus Creator/28  "MRR_ObjUpdFlg_08"
  Data Type Conversion29/1 -> Bus Creator/29  "MRR_Obj_07_08_Checksum"
  Data Type Conversion30/1 -> Bus Creator/30  "MRR_Obj_07_08_MsgCounter"
  Bus Creator/1 -> VR_ADCU_MRR_Obj_07_08_0x693FromOutData/1  "VR_ADCU_MRR_Obj_07_08_0x693FromOutData"
  VR_ADCU_MRR_Obj_07_08_0x693FromInData/1 -> CAN FD Unpack/1  "VR_ADCU_MRR_Obj_07_08_0x693FromInData"

== system ALL_JP360_DBW_V6_5_1103/MsgFromCAN/VR_ADCU_MsgFromCAN/VR_ADCU_MRR_Obj_09_10_0x694 ==
  VR_ADCU_MRR_Obj_09_10_0x694FromInData : Inport  OutDataTypeStr=Bus:CAN_FD_MESSAGE_BUS
  Bus Creator : BusCreator  Inputs=30  OutDataTypeStr=Bus:VR_ADCU_MRR_Obj_09_10_0x694  NonVirtualBus=on
  CAN FD Unpack : canfdmsglib/CAN FD Unpack  CANdbFile=HiFire_T360_P789_1R1V_Pri_Matrix_CAN_V2.3_20220810.dbc  MsgList=(none)  MsgName=MRR_Obj_09_10_0x694  ProtocolMode=CAN FD  MsgIDType=Standard (11-bit identifier)  MsgIdentifier=1684  MsgLength=32  SignalInfo={'MRR_ObjDistX_09','26','12','BE','unsigned','Standard','0','0.0625','0','0','254.9375';'MRR_ObjDistX_10','130','12','BE','unsigned','Standard','0','0.0625','0','0','254.9375';'MRR_ObjDistY_09','44','14','BE','unsigned','Standard','0','0.0078125','-64','-64','63.9922';'MRR_ObjDistY_10','148','14','BE','unsigned','Standard','0','0.0078125','-64','-64','63.9922';'MRR_ObjExistProb_09','11','5','BE','unsigned','Standard','0','0.03125','0','0','0.96875';'MRR_ObjExistProb_10','115','5','BE','unsigned','Standard','0','0.03125','0','0','0.96875';'MRR_ObjFusionCamID_09','208','8','BE','unsigned','Standard','0','1','0','0','255';'MRR_ObjFusionCamID_10','216','8','BE','unsigned','Standard','0','1','0','0','255';'MRR_ObjFusionSig_09','98','2','BE','unsigned','Standard','0','1','0','0','3';'MRR_ObjFusionSig_10','202','2','BE','unsigned','Standard','0','1','0','0','3';'MRR_ObjID_09','0','8','BE','unsigned','Standard','0','1','0','0','255';'MRR_ObjID_10','104','8','BE','unsigned','Standard','0','1','0','0','255';'MRR_ObjMovingSts_09','103','3','BE','unsigned','Standard','0','1','0','0','7';'MRR_ObjMovingSts_10','207','3','BE','unsigned','Standard','0','1','0','0','7';'MRR_ObjObstacleProb_09','22','5','BE','unsigned','Standard','0','0.03125','0','0','0.96875';'MRR_ObjObstacleProb_10','126','5','BE','unsigned','Standard','0','0.03125','0','0','0.96875';'MRR_ObjRelAccelX_09','72','10','BE','unsigned','Standard','0','0.03125','-16','-16','15.9688';'MRR_ObjRelAccelX_10','176','10','BE','unsigned','Standard','0','0.03125','-16','-16','15.9688';'MRR_ObjRelAccelY_09','94','10','BE','unsigned','Standard','0','0.03125','-16','-16','15.9688';'MRR_ObjRelAccelY_10','198','10','BE','unsigned','Standard','0','0.03125','-16','-16','15.9688';'MRR_ObjRelVelX_09','63','13','BE','unsigned','Standard','0','0.03125','-128','-128','127.9688';'MRR_ObjRelVelX_10','167','13','BE','unsigned','Standard','0','0.03125','-128','-128','127.9688';'MRR_ObjRelVelY_09','66','13','BE','unsigned','Standard','0','0.03125','-128','-128','127.9688';'MRR_ObjRelVelY_10','170','13','BE','unsigned','Standard','0','0.03125','-128','-128','127.9688';'MRR_ObjType_09','90','4','BE','unsigned','Standard','0','1','0','0','15';'MRR_ObjType_10','194','4','BE','unsigned','Standard','0','1','0','0','15';'MRR_ObjUpdFlg_09','100','3','BE','unsigned','Standard','0','1','0','0','7';'MRR_ObjUpdFlg_10','204','3','BE','unsigned','Standard','0','1','0','0','7';'MRR_Obj_09_10_Checksum','248','16','BE','unsigned','Standard','0','1','0','0','65535';'MRR_Obj_09_10_MsgCounter','232','4','BE','unsigned','Standard','0','1','0','0','15'}  IDPort=off  TimestampPort=off  ErrorPort=off  RemotePort=off  LengthPort=off  StatusPort=off  BRSPort=off  ESIPort=off  DLCPort=off  ApplyMinMax=off
      settings: SourceProductBaseCode=ME,XP,VN  DataFormat=CANdb specified signals
  Data Type Conversion{1..6,15..24} (16 alike) : DataTypeConversion  OutDataTypeStr=single  SaturateOnIntegerOverflow=off  RndMeth=Floor
  Data Type Conversion{9..10,13..14,25..28,30} (9 alike) : DataTypeConversion  OutDataTypeStr=int8  SaturateOnIntegerOverflow=off  RndMeth=Floor
  Data Type Conversion{7..8,11..12} (4 alike) : DataTypeConversion  OutDataTypeStr=uint8  SaturateOnIntegerOverflow=off  RndMeth=Floor
  Data Type Conversion29 : DataTypeConversion  OutDataTypeStr=uint16  SaturateOnIntegerOverflow=off  RndMeth=Floor
  VR_ADCU_MRR_Obj_09_10_0x694FromOutData : Outport  OutDataTypeStr=Bus:VR_ADCU_MRR_Obj_09_10_0x694
  wires:
  CAN FD Unpack/1 -> Data Type Conversion1/1
  CAN FD Unpack/2 -> Data Type Conversion2/1
  CAN FD Unpack/3 -> Data Type Conversion3/1
  CAN FD Unpack/4 -> Data Type Conversion4/1
  CAN FD Unpack/5 -> Data Type Conversion5/1
  CAN FD Unpack/6 -> Data Type Conversion6/1
  CAN FD Unpack/7 -> Data Type Conversion7/1
  CAN FD Unpack/8 -> Data Type Conversion8/1
  CAN FD Unpack/9 -> Data Type Conversion9/1
  CAN FD Unpack/10 -> Data Type Conversion10/1
  CAN FD Unpack/11 -> Data Type Conversion11/1
  CAN FD Unpack/12 -> Data Type Conversion12/1
  CAN FD Unpack/13 -> Data Type Conversion13/1
  CAN FD Unpack/14 -> Data Type Conversion14/1
  CAN FD Unpack/15 -> Data Type Conversion15/1
  CAN FD Unpack/16 -> Data Type Conversion16/1
  CAN FD Unpack/17 -> Data Type Conversion17/1
  CAN FD Unpack/18 -> Data Type Conversion18/1
  CAN FD Unpack/19 -> Data Type Conversion19/1
  CAN FD Unpack/20 -> Data Type Conversion20/1
  CAN FD Unpack/21 -> Data Type Conversion21/1
  CAN FD Unpack/22 -> Data Type Conversion22/1
  CAN FD Unpack/23 -> Data Type Conversion23/1
  CAN FD Unpack/24 -> Data Type Conversion24/1
  CAN FD Unpack/25 -> Data Type Conversion25/1
  CAN FD Unpack/26 -> Data Type Conversion26/1
  CAN FD Unpack/27 -> Data Type Conversion27/1
  CAN FD Unpack/28 -> Data Type Conversion28/1
  CAN FD Unpack/29 -> Data Type Conversion29/1
  CAN FD Unpack/30 -> Data Type Conversion30/1
  Data Type Conversion1/1 -> Bus Creator/1  "MRR_ObjDistX_09"
  Data Type Conversion2/1 -> Bus Creator/2  "MRR_ObjDistX_10"
  Data Type Conversion3/1 -> Bus Creator/3  "MRR_ObjDistY_09"
  Data Type Conversion4/1 -> Bus Creator/4  "MRR_ObjDistY_10"
  Data Type Conversion5/1 -> Bus Creator/5  "MRR_ObjExistProb_09"
  Data Type Conversion6/1 -> Bus Creator/6  "MRR_ObjExistProb_10"
  Data Type Conversion7/1 -> Bus Creator/7  "MRR_ObjFusionCamID_09"
  Data Type Conversion8/1 -> Bus Creator/8  "MRR_ObjFusionCamID_10"
  Data Type Conversion9/1 -> Bus Creator/9  "MRR_ObjFusionSig_09"
  Data Type Conversion10/1 -> Bus Creator/10  "MRR_ObjFusionSig_10"
  Data Type Conversion11/1 -> Bus Creator/11  "MRR_ObjID_09"
  Data Type Conversion12/1 -> Bus Creator/12  "MRR_ObjID_10"
  Data Type Conversion13/1 -> Bus Creator/13  "MRR_ObjMovingSts_09"
  Data Type Conversion14/1 -> Bus Creator/14  "MRR_ObjMovingSts_10"
  Data Type Conversion15/1 -> Bus Creator/15  "MRR_ObjObstacleProb_09"
  Data Type Conversion16/1 -> Bus Creator/16  "MRR_ObjObstacleProb_10"
  Data Type Conversion17/1 -> Bus Creator/17  "MRR_ObjRelAccelX_09"
  Data Type Conversion18/1 -> Bus Creator/18  "MRR_ObjRelAccelX_10"
  Data Type Conversion19/1 -> Bus Creator/19  "MRR_ObjRelAccelY_09"
  Data Type Conversion20/1 -> Bus Creator/20  "MRR_ObjRelAccelY_10"
  Data Type Conversion21/1 -> Bus Creator/21  "MRR_ObjRelVelX_09"
  Data Type Conversion22/1 -> Bus Creator/22  "MRR_ObjRelVelX_10"
  Data Type Conversion23/1 -> Bus Creator/23  "MRR_ObjRelVelY_09"
  Data Type Conversion24/1 -> Bus Creator/24  "MRR_ObjRelVelY_10"
  Data Type Conversion25/1 -> Bus Creator/25  "MRR_ObjType_09"
  Data Type Conversion26/1 -> Bus Creator/26  "MRR_ObjType_10"
  Data Type Conversion27/1 -> Bus Creator/27  "MRR_ObjUpdFlg_09"
  Data Type Conversion28/1 -> Bus Creator/28  "MRR_ObjUpdFlg_10"
  Data Type Conversion29/1 -> Bus Creator/29  "MRR_Obj_09_10_Checksum"
  Data Type Conversion30/1 -> Bus Creator/30  "MRR_Obj_09_10_MsgCounter"
  Bus Creator/1 -> VR_ADCU_MRR_Obj_09_10_0x694FromOutData/1  "VR_ADCU_MRR_Obj_09_10_0x694FromOutData"
  VR_ADCU_MRR_Obj_09_10_0x694FromInData/1 -> CAN FD Unpack/1  "VR_ADCU_MRR_Obj_09_10_0x694FromInData"

== system ALL_JP360_DBW_V6_5_1103/MsgFromCAN/VR_ADCU_MsgFromCAN/VR_ADCU_MRR_Obj_11_12_0x695 ==
  VR_ADCU_MRR_Obj_11_12_0x695FromInData : Inport  OutDataTypeStr=Bus:CAN_FD_MESSAGE_BUS
  Bus Creator : BusCreator  Inputs=30  OutDataTypeStr=Bus:VR_ADCU_MRR_Obj_11_12_0x695  NonVirtualBus=on
  CAN FD Unpack : canfdmsglib/CAN FD Unpack  CANdbFile=HiFire_T360_P789_1R1V_Pri_Matrix_CAN_V2.3_20220810.dbc  MsgList=(none)  MsgName=MRR_Obj_11_12_0x695  ProtocolMode=CAN FD  MsgIDType=Standard (11-bit identifier)  MsgIdentifier=1685  MsgLength=32  SignalInfo={'MRR_ObjDistX_11','26','12','BE','unsigned','Standard','0','0.0625','0','0','254.9375';'MRR_ObjDistX_12','130','12','BE','unsigned','Standard','0','0.0625','0','0','254.9375';'MRR_ObjDistY_11','44','14','BE','unsigned','Standard','0','0.0078125','-64','-64','63.9922';'MRR_ObjDistY_12','148','14','BE','unsigned','Standard','0','0.0078125','-64','-64','63.9922';'MRR_ObjExistProb_11','11','5','BE','unsigned','Standard','0','0.03125','0','0','0.96875';'MRR_ObjExistProb_12','115','5','BE','unsigned','Standard','0','0.03125','0','0','0.96875';'MRR_ObjFusionCamID_11','208','8','BE','unsigned','Standard','0','1','0','0','255';'MRR_ObjFusionCamID_12','216','8','BE','unsigned','Standard','0','1','0','0','255';'MRR_ObjFusionSig_11','98','2','BE','unsigned','Standard','0','1','0','0','3';'MRR_ObjFusionSig_12','202','2','BE','unsigned','Standard','0','1','0','0','3';'MRR_ObjID_11','0','8','BE','unsigned','Standard','0','1','0','0','255';'MRR_ObjID_12','104','8','BE','unsigned','Standard','0','1','0','0','255';'MRR_ObjMovingSts_11','103','3','BE','unsigned','Standard','0','1','0','0','7';'MRR_ObjMovingSts_12','207','3','BE','unsigned','Standard','0','1','0','0','7';'MRR_ObjObstacleProb_11','22','5','BE','unsigned','Standard','0','0.03125','0','0','0.96875';'MRR_ObjObstacleProb_12','126','5','BE','unsigned','Standard','0','0.03125','0','0','0.96875';'MRR_ObjRelAccelX_11','72','10','BE','unsigned','Standard','0','0.03125','-16','-16','15.9688';'MRR_ObjRelAccelX_12','176','10','BE','unsigned','Standard','0','0.03125','-16','-16','15.9688';'MRR_ObjRelAccelY_11','94','10','BE','unsigned','Standard','0','0.03125','-16','-16','15.9688';'MRR_ObjRelAccelY_12','198','10','BE','unsigned','Standard','0','0.03125','-16','-16','15.9688';'MRR_ObjRelVelX_11','63','13','BE','unsigned','Standard','0','0.03125','-128','-128','127.9688';'MRR_ObjRelVelX_12','167','13','BE','unsigned','Standard','0','0.03125','-128','-128','127.9688';'MRR_ObjRelVelY_11','66','13','BE','unsigned','Standard','0','0.03125','-128','-128','127.9688';'MRR_ObjRelVelY_12','170','13','BE','unsigned','Standard','0','0.03125','-128','-128','127.9688';'MRR_ObjType_11','90','4','BE','unsigned','Standard','0','1','0','0','15';'MRR_ObjType_12','194','4','BE','unsigned','Standard','0','1','0','0','15';'MRR_ObjUpdFlg_11','100','3','BE','unsigned','Standard','0','1','0','0','7';'MRR_ObjUpdFlg_12','204','3','BE','unsigned','Standard','0','1','0','0','7';'MRR_Obj_11_12_Checksum','248','16','BE','unsigned','Standard','0','1','0','0','65535';'MRR_Obj_11_12_MsgCounter','232','4','BE','unsigned','Standard','0','1','0','0','15'}  IDPort=off  TimestampPort=off  ErrorPort=off  RemotePort=off  LengthPort=off  StatusPort=off  BRSPort=off  ESIPort=off  DLCPort=off  ApplyMinMax=off
      settings: SourceProductBaseCode=ME,XP,VN  DataFormat=CANdb specified signals
  Data Type Conversion{1..6,15..24} (16 alike) : DataTypeConversion  OutDataTypeStr=single  SaturateOnIntegerOverflow=off  RndMeth=Floor
  Data Type Conversion{9..10,13..14,25..28,30} (9 alike) : DataTypeConversion  OutDataTypeStr=int8  SaturateOnIntegerOverflow=off  RndMeth=Floor
  Data Type Conversion{7..8,11..12} (4 alike) : DataTypeConversion  OutDataTypeStr=uint8  SaturateOnIntegerOverflow=off  RndMeth=Floor
  Data Type Conversion29 : DataTypeConversion  OutDataTypeStr=uint16  SaturateOnIntegerOverflow=off  RndMeth=Floor
  VR_ADCU_MRR_Obj_11_12_0x695FromOutData : Outport  OutDataTypeStr=Bus:VR_ADCU_MRR_Obj_11_12_0x695
  wires:
  CAN FD Unpack/1 -> Data Type Conversion1/1
  CAN FD Unpack/2 -> Data Type Conversion2/1
  CAN FD Unpack/3 -> Data Type Conversion3/1
  CAN FD Unpack/4 -> Data Type Conversion4/1
  CAN FD Unpack/5 -> Data Type Conversion5/1
  CAN FD Unpack/6 -> Data Type Conversion6/1
  CAN FD Unpack/7 -> Data Type Conversion7/1
  CAN FD Unpack/8 -> Data Type Conversion8/1
  CAN FD Unpack/9 -> Data Type Conversion9/1
  CAN FD Unpack/10 -> Data Type Conversion10/1
  CAN FD Unpack/11 -> Data Type Conversion11/1
  CAN FD Unpack/12 -> Data Type Conversion12/1
  CAN FD Unpack/13 -> Data Type Conversion13/1
  CAN FD Unpack/14 -> Data Type Conversion14/1
  CAN FD Unpack/15 -> Data Type Conversion15/1
  CAN FD Unpack/16 -> Data Type Conversion16/1
  CAN FD Unpack/17 -> Data Type Conversion17/1
  CAN FD Unpack/18 -> Data Type Conversion18/1
  CAN FD Unpack/19 -> Data Type Conversion19/1
  CAN FD Unpack/20 -> Data Type Conversion20/1
  CAN FD Unpack/21 -> Data Type Conversion21/1
  CAN FD Unpack/22 -> Data Type Conversion22/1
  CAN FD Unpack/23 -> Data Type Conversion23/1
  CAN FD Unpack/24 -> Data Type Conversion24/1
  CAN FD Unpack/25 -> Data Type Conversion25/1
  CAN FD Unpack/26 -> Data Type Conversion26/1
  CAN FD Unpack/27 -> Data Type Conversion27/1
  CAN FD Unpack/28 -> Data Type Conversion28/1
  CAN FD Unpack/29 -> Data Type Conversion29/1
  CAN FD Unpack/30 -> Data Type Conversion30/1
  Data Type Conversion1/1 -> Bus Creator/1  "MRR_ObjDistX_11"
  Data Type Conversion2/1 -> Bus Creator/2  "MRR_ObjDistX_12"
  Data Type Conversion3/1 -> Bus Creator/3  "MRR_ObjDistY_11"
  Data Type Conversion4/1 -> Bus Creator/4  "MRR_ObjDistY_12"
  Data Type Conversion5/1 -> Bus Creator/5  "MRR_ObjExistProb_11"
  Data Type Conversion6/1 -> Bus Creator/6  "MRR_ObjExistProb_12"
  Data Type Conversion7/1 -> Bus Creator/7  "MRR_ObjFusionCamID_11"
  Data Type Conversion8/1 -> Bus Creator/8  "MRR_ObjFusionCamID_12"
  Data Type Conversion9/1 -> Bus Creator/9  "MRR_ObjFusionSig_11"
  Data Type Conversion10/1 -> Bus Creator/10  "MRR_ObjFusionSig_12"
  Data Type Conversion11/1 -> Bus Creator/11  "MRR_ObjID_11"
  Data Type Conversion12/1 -> Bus Creator/12  "MRR_ObjID_12"
  Data Type Conversion13/1 -> Bus Creator/13  "MRR_ObjMovingSts_11"
  Data Type Conversion14/1 -> Bus Creator/14  "MRR_ObjMovingSts_12"
  Data Type Conversion15/1 -> Bus Creator/15  "MRR_ObjObstacleProb_11"
  Data Type Conversion16/1 -> Bus Creator/16  "MRR_ObjObstacleProb_12"
  Data Type Conversion17/1 -> Bus Creator/17  "MRR_ObjRelAccelX_11"
  Data Type Conversion18/1 -> Bus Creator/18  "MRR_ObjRelAccelX_12"
  Data Type Conversion19/1 -> Bus Creator/19  "MRR_ObjRelAccelY_11"
  Data Type Conversion20/1 -> Bus Creator/20  "MRR_ObjRelAccelY_12"
  Data Type Conversion21/1 -> Bus Creator/21  "MRR_ObjRelVelX_11"
  Data Type Conversion22/1 -> Bus Creator/22  "MRR_ObjRelVelX_12"
  Data Type Conversion23/1 -> Bus Creator/23  "MRR_ObjRelVelY_11"
  Data Type Conversion24/1 -> Bus Creator/24  "MRR_ObjRelVelY_12"
  Data Type Conversion25/1 -> Bus Creator/25  "MRR_ObjType_11"
  Data Type Conversion26/1 -> Bus Creator/26  "MRR_ObjType_12"
  Data Type Conversion27/1 -> Bus Creator/27  "MRR_ObjUpdFlg_11"
  Data Type Conversion28/1 -> Bus Creator/28  "MRR_ObjUpdFlg_12"
  Data Type Conversion29/1 -> Bus Creator/29  "MRR_Obj_11_12_Checksum"
  Data Type Conversion30/1 -> Bus Creator/30  "MRR_Obj_11_12_MsgCounter"
  Bus Creator/1 -> VR_ADCU_MRR_Obj_11_12_0x695FromOutData/1  "VR_ADCU_MRR_Obj_11_12_0x695FromOutData"
  VR_ADCU_MRR_Obj_11_12_0x695FromInData/1 -> CAN FD Unpack/1  "VR_ADCU_MRR_Obj_11_12_0x695FromInData"
